simulink library "filter_library"  (R2018a)
settings: Solver=VariableStepAuto  StartTime=0.0  StopTime=10.0  RelTol=1e-3
undefined symbols (not defined in the file or in its folder): a, b, c
libraries: hdlsllib x1
settings Model: Creator=Orion  LastModifiedBy=Orion

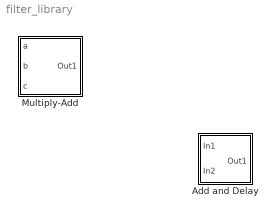
== system filter_library ==
  Add and Delay : Subsystem  mask{Inputs=++}
      mask prompts: Inputs "Simulink:blkprm_prompts:SumListofSigns"
      mask TypeOptions Inputs: Add/Inputs
      mask DialogControl Inputs Prompt: List of signs:
      mask Display:
      | fprintf('a+b')
      | port_label('input', 1, 'a')
      | port_label('input', 2, 'b')
  Multiply-Add : Subsystem
      mask Display:
      | fprintf('(a*b)+c')
      | port_label('input', 1, 'a')
      | port_label('input', 2, 'b')
      | port_label('input', 3, 'c')

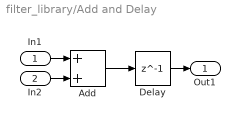
== system filter_library/Add and Delay ==
  In1 : Inport
  In2 : Inport  Port=2
  Add : Sum  OutDataTypeStr=Inherit: Inherit via back propagation
  Delay : Delay  DelayLength=1  InitialCondition=0
  Out1 : Outport
  wires:
  Add/1 -> Delay/1
  In2/1 -> Add/2
  In1/1 -> Add/1
  Delay/1 -> Out1/1

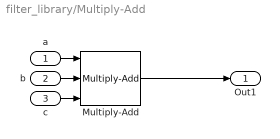
== system filter_library/Multiply-Add ==
  a : Inport
  b : Inport  Port=2
  c : Inport  Port=3
  Multiply-Add : hdlsllib/HDL Operations/Multiply-Add  Function=c+(a.*b)  datatype=Inherit: Inherit via back propagation  DoSatur=off  FMA=off
      settings: SourceProductName=HDL Coder  SourceProductBaseCode=HD
  Out1 : Outport
  wires:
  c/1 -> Multiply-Add/3
  a/1 -> Multiply-Add/1
  b/1 -> Multiply-Add/2
  Multiply-Add/1 -> Out1/1
